simulink model "req5"  (R2019a)
settings: Solver=FixedStepAuto  StartTime=0.0  StopTime=100  RelTol=1e-3
settings Model: Creator=e40014285  LastModifiedBy=e40014285
settings ConfigComp: CovEnable=on  CovScope=ReferencedModels  RecordCoverage=on

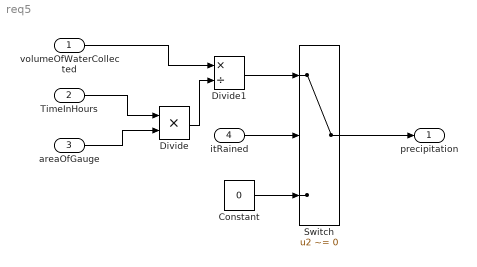
== system req5 ==
  volumeOfWaterCollected : Inport
  TimeInHours : Inport  Port=2
  areaOfGauge : Inport  Port=3
  itRained : Inport  Port=4
  Constant : Constant  Value=0
  Divide : Product  Inputs=**
  Divide1 : Product  Inputs=*/
  Switch : Switch  Criteria=u2 ~= 0  Threshold=~0
  precipitation : Outport
  wires:
  areaOfGauge/1 -> Divide/2
  TimeInHours/1 -> Divide/1
  volumeOfWaterCollected/1 -> Divide1/1
  Divide/1 -> Divide1/2
  Divide1/1 -> Switch/1
  Switch/1 -> precipitation/1
  itRained/1 -> Switch/2
  Constant/1 -> Switch/3
